simulink model "Pass_Time_Tester"  (R2018b)
settings: Solver=FixedStepDiscrete  StartTime=0.0  StopTime=5700000  FixedStep=1  RelTol=1e-3
values from neighbouring files (symbols this model uses):
  simParams = struct    [rwa_power_model.m]
undefined symbols (not defined in the file or in its folder): clock_lib, DiscIntNeverNeededParam, fswParams
libraries: sgp4_lib_fsw x1, target_groundpass_lib x1, time_coord_rotations_lib x1
settings Model: Creator=Nick's PC  LastModifiedBy=Nick's PC

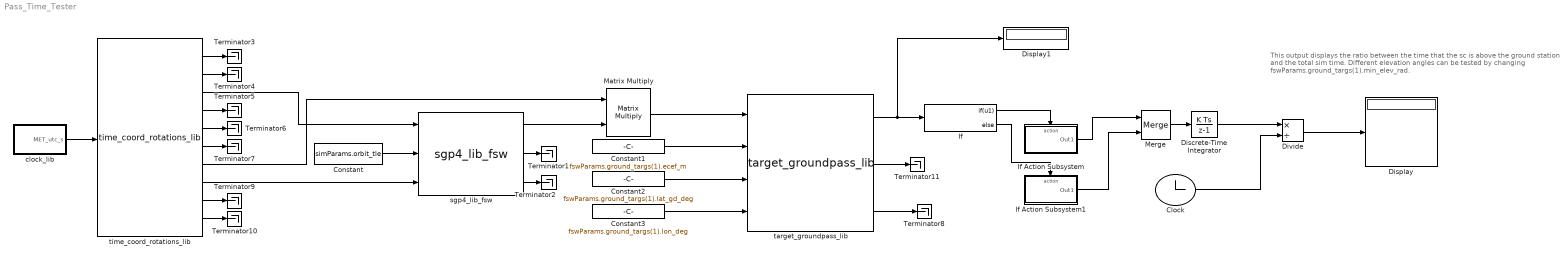
== system Pass_Time_Tester ==
  note: This output displays the ratio between the time that the sc is above the ground
      | station and the total sim time. Different elevation angles can be tested by changing
      | fswParams.ground_targs(1).min_elev_rad.
  Clock : Clock
  Constant : Constant  Value=simParams.orbit_tle
  Constant1 : Constant  Value=fswParams.ground_targs(1).ecef_m
  Constant2 : Constant  Value=fswParams.ground_targs(1).lat_gd_deg
  Constant3 : Constant  Value=fswParams.ground_targs(1).lon_deg
  Discrete-Time Integrator : DiscreteIntegrator  SampleTime=-1  ICPrevOutput=DiscIntNeverNeededParam  ICPrevScaledInput=DiscIntNeverNeededParam
  Display : Display
  Display1 : Display
  Divide : Product  Inputs=*/
  If : If  IfExpression=u1
  If Action Subsystem : Subsystem  TreatAsAtomicUnit=on
  If Action Subsystem1 : Subsystem  TreatAsAtomicUnit=on
  Matrix Multiply : Product  Multiplication=Matrix(*)
  Merge : Merge
  Terminator{1..11} (11 alike) : Terminator
  clock_lib : Subsystem  AncestorBlock=clock_lib/clock_lib
  sgp4_lib_fsw : sgp4_lib_fsw/sgp4_lib_fsw  SystemSampleTime=-1
  target_groundpass_lib : target_groundpass_lib/target_groundpass_lib  id=1
  "time_coord_rotations_lib " : time_coord_rotations_lib/time_coord_rotations_lib    time_offset=fswParams.sensors.time_offset
  wires:
  "time_coord_rotations_lib "/6 -> Terminator7/1
  Clock/1 -> Divide/2
  "time_coord_rotations_lib "/10 -> Terminator10/1
  "time_coord_rotations_lib "/4 -> Terminator5/1
  "time_coord_rotations_lib "/5 -> Terminator6/1
  "time_coord_rotations_lib "/8 -> sgp4_lib_fsw/3
  "time_coord_rotations_lib "/2 -> Terminator4/1
  "time_coord_rotations_lib "/1 -> Terminator3/1
  "time_coord_rotations_lib "/3 -> sgp4_lib_fsw/1
  "time_coord_rotations_lib "/9 -> Terminator9/1
  Constant/1 -> sgp4_lib_fsw/2
  "time_coord_rotations_lib "/7 -> Matrix Multiply/1
  sgp4_lib_fsw/1 -> Matrix Multiply/2
  sgp4_lib_fsw/2 -> Terminator1/1
  sgp4_lib_fsw/3 -> Terminator2/1
  Constant1/1 -> target_groundpass_lib/2
  Constant3/1 -> target_groundpass_lib/4
  Constant2/1 -> target_groundpass_lib/3
  Matrix Multiply/1 -> target_groundpass_lib/1
  target_groundpass_lib/3 -> Terminator8/1
  target_groundpass_lib/2 -> Terminator11/1
  target_groundpass_lib/1 -> Display1/1, If/1
  Discrete-Time Integrator/1 -> Divide/1
  Divide/1 -> Display/1
  If/1 -> If Action Subsystem/Action
  If/2 -> If Action Subsystem1/Action
  Merge/1 -> Discrete-Time Integrator/1
  If Action Subsystem1/1(Out1) -> Merge/2
  If Action Subsystem/1(Out1) -> Merge/1
  clock_lib/1(MET_utc_s) -> "time_coord_rotations_lib "/1

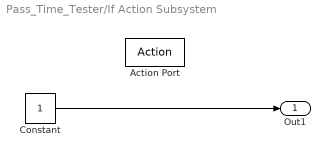
== system Pass_Time_Tester/If Action Subsystem ==
  Action Port : ActionPort  ActionType=then
  Constant : Constant
  Out1 : Outport
  wires:
  Constant/1 -> Out1/1

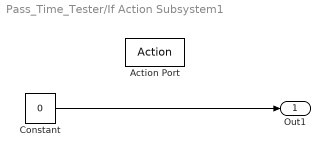
== system Pass_Time_Tester/If Action Subsystem1 ==
  Action Port : ActionPort  ActionType=else
  Constant : Constant  Value=0
  Out1 : Outport
  wires:
  Constant/1 -> Out1/1

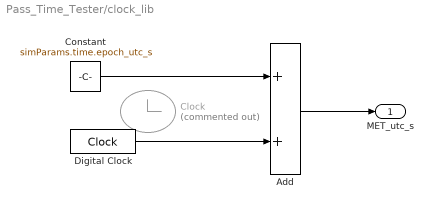
== system Pass_Time_Tester/clock_lib ==
  Add : Sum
  Clock : Clock  Commented=on
  Constant : Constant  Value=simParams.time.epoch_utc_s
  Digital Clock : DigitalClock
  MET_utc_s : Outport
  wires:
  Add/1 -> MET_utc_s/1
  Digital Clock/1 -> Add/2
  Constant/1 -> Add/1
